simulink model "tf_mcp_lub_oil"  (R2020a)
settings: Solver=FixedStepAuto  StartTime=0.0  StopTime=10.0  RelTol=1e-3
model workspace (MAT data in the model file):
  max_mcp_lub_oil_temp = 80
  min_mcp_lub_oil_press = 1.2
undefined symbols (not defined in the file): mcp_nominal_rotation
libraries: simulink x1
settings Model: Creator=ToT_IPMS_03  LastModifiedBy=suina
settings OptimizationCC: DefaultParameterBehavior=Inlined  EnhancedBackFolding=on  PassReuseOutputArgsAs=Individual arguments  ZeroExternalMemoryAtStartup=off  ZeroInternalMemoryAtStartup=off  OptimizeBlockOrder=speed  DifferentSizesBufferReuse=on  OptimizationCustomize=off  EfficientTunableParamExpr=on
settings DebuggingCC: ParameterTunabilityLossMsg=error
settings SFSimCC: MATLABDynamicMemAlloc=off
settings RTWCC: SystemTargetFile=ert.tlc  TemplateMakefile=ert_default_tmf
settings CodeAppCC: ForceParamTrailComments=on  IgnoreCustomStorageClasses=off  OperatorAnnotations=on  SimulinkDataObjDesc=on  SFDataObjDesc=on  InsertBlockDesc=on
settings ERTTargetCC: TargetLangStandard=C99 (ISO)  GenerateSampleERTMain=on  InlinedParameterPlacement=NonHierarchical  ERTCustomFileTemplate=example_file_process.tlc

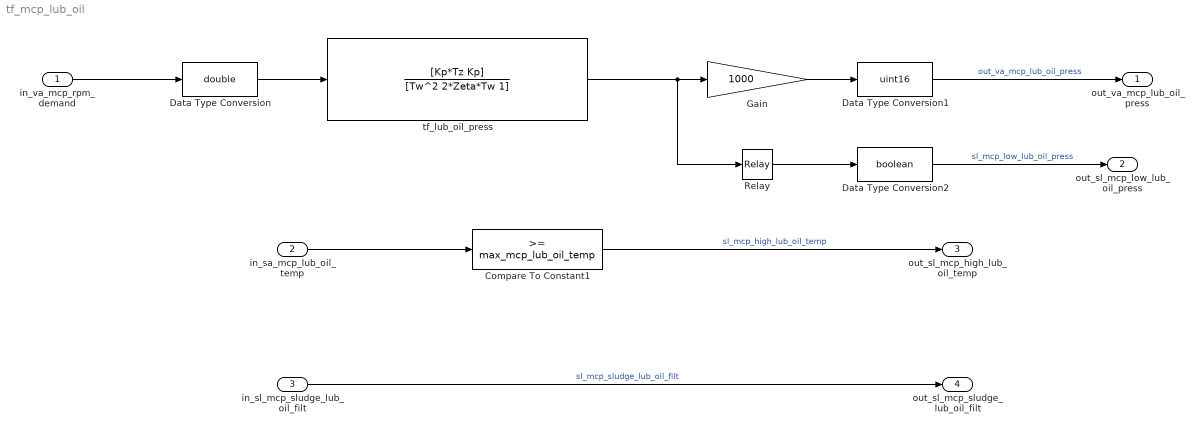
== system tf_mcp_lub_oil ==
  in_va_mcp_rpm_demand : Inport  OutMin=[0]  OutMax=[mcp_nominal_rotation]  OutDataTypeStr=uint16  Unit=%  PortDimensions=1  SampleTime=0
  in_sa_mcp_lub_oil_temp : Inport  Port=2  OutMin=[0]  OutMax=[100]  OutDataTypeStr=uint16  Unit=°C
  in_sl_mcp_sludge_lub_oil_filt : Inport  Port=3  OutDataTypeStr=boolean
  Compare To Constant1 : simulink/Logic and Bit Operations/Compare To Constant  relop=>=  const=max_mcp_lub_oil_temp  OutDataTypeStr=boolean
  Data Type Conversion : DataTypeConversion  OutDataTypeStr=double
  Data Type Conversion1 : DataTypeConversion  OutDataTypeStr=uint16  RndMeth=Nearest
  Data Type Conversion2 : DataTypeConversion  OutDataTypeStr=boolean
  Gain : Gain  Gain=1000
  Relay : Relay  OnSwitchValue=min_mcp_lub_oil_press+0.1  OffSwitchValue=min_mcp_lub_oil_press-0.1  OnOutputValue=0  OffOutputValue=1
  tf_lub_oil_press : TransferFcn  Numerator=[Kp*Tz Kp]  Denominator=[Tw^2 2*Zeta*Tw 1]  mask{Kp=0.0042, Tz=13.563, Tw=7.2155, Zeta=0.97827, Td=0}
  out_va_mcp_lub_oil_press : Outport  OutMin=[0]  OutMax=[100]  OutDataTypeStr=uint16  Unit=MPa  PortDimensions=1  SampleTime=0
  out_sl_mcp_low_lub_oil_press : Outport  Port=2  OutDataTypeStr=boolean
  out_sl_mcp_high_lub_oil_temp : Outport  Port=3  OutMin=[0]  OutMax=[1]  OutDataTypeStr=boolean
  out_sl_mcp_sludge_lub_oil_filt : Outport  Port=4
  wires:
  in_va_mcp_rpm_demand/1 -> Data Type Conversion/1
  Data Type Conversion1/1 -> out_va_mcp_lub_oil_press/1  "out_va_mcp_lub_oil_press"
  Compare To Constant1/1 -> out_sl_mcp_high_lub_oil_temp/1  "sl_mcp_high_lub_oil_temp"
  in_sa_mcp_lub_oil_temp/1 -> Compare To Constant1/1
  in_sl_mcp_sludge_lub_oil_filt/1 -> out_sl_mcp_sludge_lub_oil_filt/1  "sl_mcp_sludge_lub_oil_filt"
  Relay/1 -> Data Type Conversion2/1
  Data Type Conversion/1 -> tf_lub_oil_press/1
  tf_lub_oil_press/1 -> Relay/1, Gain/1
  Gain/1 -> Data Type Conversion1/1
  Data Type Conversion2/1 -> out_sl_mcp_low_lub_oil_press/1  "sl_mcp_low_lub_oil_press"
